simulink model "testbench_ultrasonic_object"  (R2015a)
settings: Solver=ode45  StartTime=0.0  StopTime=10.0  RelTol=1e-3
libraries: simulink x2, legoev3lib x2
settings Model: Creator=USER  LastModifiedBy=USER

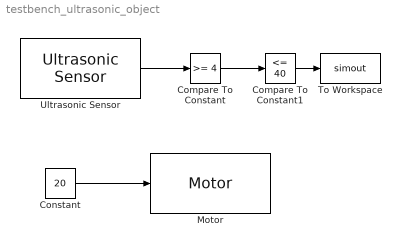
== system testbench_ultrasonic_object ==
  Compare To Constant : simulink/Logic and Bit Operations/Compare To Constant  relop=>=  const=4  OutDataTypeStr=uint8
  Compare To Constant1 : simulink/Logic and Bit Operations/Compare To Constant  relop=<=  const=40  OutDataTypeStr=uint8
  Constant : Constant  Value=20
  Motor : legoev3lib/Motor  sportNumber=A  sstopAction=Brake
  To Workspace : ToWorkspace  VariableName=simout  SampleTime=-1
      settings: Save2DSignal=2-D array (concatenate along first dimension)
  Ultrasonic Sensor : legoev3lib/Ultrasonic Sensor  PortNumber=1  sampleTime=0.1
  wires:
  Ultrasonic Sensor/1 -> Compare To Constant/1
  Compare To Constant/1 -> Compare To Constant1/1
  Compare To Constant1/1 -> To Workspace/1
  Constant/1 -> Motor/1
